simulink library "periodicCtrlExp"  (R2020a)
settings: Solver=VariableStepAuto  StartTime=0.0  StopTime=10.0  RelTol=1e-3
undefined symbols (not defined in the file or in its folder): fltCtrl, initializeBussesFromBlock
libraries: dspsigops x2, filteredPIDController_ul x2
settings Model: Creator=jcreed2  LastModifiedBy=andre

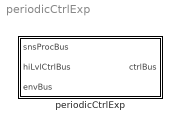
== system periodicCtrlExp ==
  periodicCtrlExp : Subsystem  LoadFcn=initializeBussesFromBlock(gcb)  InitFcn=initializeBussesFromBlock(gcb)  mask{fltCtrl=fltCtrl}
      mask prompts: fltCtrl "Controller Model"

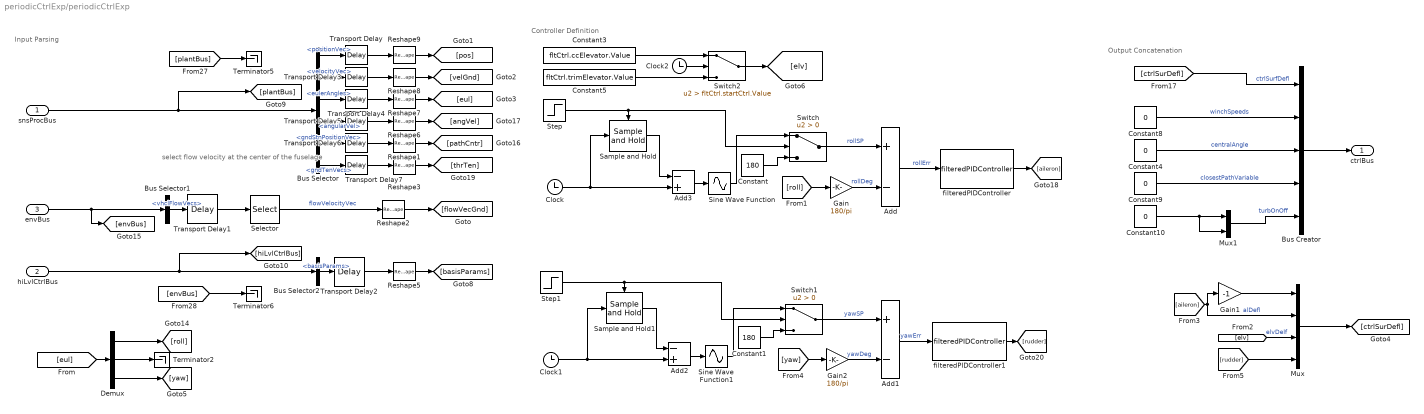
== system periodicCtrlExp/periodicCtrlExp ==
  note: Controller Definition
  note: select flow velocity at the center of the fuselage
  note: Input Parsing
  note: Output Concatenation
  snsProcBus : Inport  OutDataTypeStr=Bus: sensorsProcessingBus
  hiLvlCtrlBus : Inport  Port=2  OutDataTypeStr=Bus: hiLvlCtrlBus
  envBus : Inport  Port=3  OutDataTypeStr=Bus: envBus
  Add : Sum  Inputs=+-
  Add1 : Sum  Inputs=+-
  Add2 : Sum  Inputs=-+
  Add3 : Sum  Inputs=-+
  Bus Creator : BusCreator  Inputs=5  OutDataTypeStr=Bus: fltCtrlBus
      settings: InheritFromInputs=off
  Bus Selector : BusSelector  OutputSignals=positionVec,velocityVec,eulerAngles,angularVel,gndStnPositionVec,gndTenVecs
  Bus Selector1 : BusSelector  OutputSignals=vhclFlowVecs
  Bus Selector2 : BusSelector  OutputSignals=basisParams
  Clock : Clock
  Clock1 : Clock
  Clock2 : Clock
  Constant : Constant  Value=180
  Constant1 : Constant  Value=180
  Constant{4,8..10} (4 alike) : Constant  Value=0
  Constant3 : Constant  Value=fltCtrl.ccElevator.Value
  Constant5 : Constant  Value=fltCtrl.trimElevator.Value
  Demux : Demux  Outputs=3
  Gain : Gain  Gain=180/pi
  Gain1 : Gain  Gain=-1
  Gain2 : Gain  Gain=180/pi
  Mux : Mux
  Mux1 : Mux  Inputs=2
  Reshape{1..3,5..9} (8 alike) : Reshape  OutputDimensionality=Column vector (2-D)
  Sample and Hold : dspsigops/Sample and Hold  trig=Rising edge  initCond=0  latchinput=off
  Sample and Hold1 : dspsigops/Sample and Hold  trig=Rising edge  initCond=0  latchinput=off
  Selector : Selector  NumberOfDimensions=2  InputPortWidth=3  IndexOptions=Select all,Index vector (dialog)  Indices=[1 3],5  OutputSizes=1,1
  Sine Wave Function : Sin  TimeSource=Use external signal  Amplitude=fltCtrl.rollAmp.Value  Bias=180  Frequency=fltCtrl.frequency.Value  Phase=pi  SampleTime=0
  Sine Wave Function1 : Sin  TimeSource=Use external signal  Amplitude=fltCtrl.yawAmp.Value  Bias=180  Frequency=fltCtrl.frequency.Value  Phase=2/10*pi  SampleTime=0
  Step : Step  Time=fltCtrl.startCtrl.Value  SampleTime=0
  Step1 : Step  Time=fltCtrl.startCtrl.Value  SampleTime=0
  Switch : Switch  Criteria=u2 > Threshold
  Switch1 : Switch  Criteria=u2 > Threshold
  Switch2 : Switch  Criteria=u2 > Threshold  Threshold=fltCtrl.startCtrl.Value
  Terminator2 : Terminator
  Terminator5 : Terminator
  Terminator6 : Terminator
  Transport Delay{,1..7} (8 alike) : TransportDelay  DelayTime=.060
  filteredPIDController : filteredPIDController_ul/filteredPIDController  kp=fltCtrl.rollCtrl.kp.Value  ki=fltCtrl.rollCtrl.ki.Value  kd=fltCtrl.rollCtrl.kd.Value  Value=fltCtrl.rollCtrl.tau.Value  externalReset=none
  filteredPIDController1 : filteredPIDController_ul/filteredPIDController  kp=fltCtrl.yawCtrl.kp.Value  ki=fltCtrl.yawCtrl.ki.Value  kd=fltCtrl.yawCtrl.kd.Value  Value=fltCtrl.yawCtrl.tau.Value  externalReset=none
  ctrlBus : Outport  OutDataTypeStr=Bus: fltCtrlBus  VectorParamsAs1DForOutWhenUnconnected=off
  wires:
  Reshape1/1 -> [pathCntr]
  Reshape9/1 -> [pos]
  Bus Selector/5 -> Transport Delay6/1  "<gndStnPositionVec>"
  Bus Selector/3 -> Transport Delay4/1  "<eulerAngles>"
  Demux/2 -> Terminator2/1
  Gain1/1 -> Mux/1
  [envBus] -> Terminator6/1
  Reshape3/1 -> [thrTen]
  [rudder] -> Mux/4
  Constant5/1 -> Switch2/3
  Reshape5/1 -> [basisParams]
  envBus/1 -> [envBus], Bus Selector1/1
  Bus Creator/1 -> ctrlBus/1
  Bus Selector/1 -> Transport Delay/1  "<positionVec>"
  Constant8/1 -> Bus Creator/2  "winchSpeeds"
  Bus Selector/4 -> Transport Delay5/1  "<angularVel>"
  Reshape6/1 -> [angVel]
  Bus Selector2/1 -> Transport Delay2/1  "<basisParams>"
  Bus Selector/2 -> Transport Delay3/1  "<velocityVec>"
  [aileron] -> Mux/2, Gain1/1  "alDefl"
  Reshape2/1 -> [flowVecGnd]
  [ctrlSurDefl] -> Bus Creator/1  "ctrlSurfDefl"
  [elv] -> Mux/3  "elvDelf"
  [plantBus] -> Terminator5/1
  Reshape7/1 -> [eul]
  Selector/1 -> Reshape2/1  "flowVelocityVec"
  [eul] -> Demux/1
  Bus Selector/6 -> Transport Delay7/1  "<gndTenVecs>"
  Demux/1 -> [roll]
  Demux/3 -> [yaw]
  Reshape8/1 -> [velGnd]
  Bus Selector1/1 -> Transport Delay1/1  "<vhclFlowVecs>"
  [roll] -> Gain/1
  Add/1 -> filteredPIDController/1  "rollErr"
  Gain/1 -> Add/2  "rollDeg"
  filteredPIDController/1 -> [aileron]
  filteredPIDController1/1 -> [rudder]
  Clock/1 -> Add3/2, Sample and Hold/1
  Mux/1 -> [ctrlSurDefl]
  Clock2/1 -> Switch2/2
  Switch2/1 -> [elv]
  Constant3/1 -> Switch2/1
  Sample and Hold/1 -> Add3/1
  Add3/1 -> Sine Wave Function/1
  Sine Wave Function/1 -> Switch/1
  Step/1 -> Switch/2, Sample and Hold/Trigger
  Constant/1 -> Switch/3
  Switch/1 -> Add/1  "rollSP"
  Constant4/1 -> Bus Creator/3  "centralAngle"
  Constant9/1 -> Bus Creator/4  "closestPathVariable"
  Constant10/1 -> Mux1/2, Mux1/1
  Mux1/1 -> Bus Creator/5  "turbOnOff"
  Step1/1 -> Sample and Hold1/Trigger, Switch1/2
  Constant1/1 -> Switch1/3
  Switch1/1 -> Add1/1  "yawSP"
  Sine Wave Function1/1 -> Switch1/1
  Add2/1 -> Sine Wave Function1/1
  Gain2/1 -> Add1/2  "yawDeg"
  [yaw] -> Gain2/1
  Sample and Hold1/1 -> Add2/1
  Clock1/1 -> Sample and Hold1/1, Add2/2
  Add1/1 -> filteredPIDController1/1  "yawErr"
  snsProcBus/1 -> Bus Selector/1, [plantBus]
  Transport Delay1/1 -> Selector/1
  hiLvlCtrlBus/1 -> [hiLvlCtrlBus], Bus Selector2/1
  Transport Delay/1 -> Reshape9/1
  Transport Delay3/1 -> Reshape8/1
  Transport Delay4/1 -> Reshape7/1
  Transport Delay5/1 -> Reshape6/1
  Transport Delay6/1 -> Reshape1/1
  Transport Delay7/1 -> Reshape3/1
  Transport Delay2/1 -> Reshape5/1
